simulink library "libturbines"  (Simulink 7.9)
settings: Solver=ode45  StartTime=0.0  StopTime=10.0  RelTol=1e-3
undefined symbols (not defined in the file): DiscIntNeverNeededParam
libraries: simulink x2
settings Model: Creator=grunnet  LastModifiedBy=mikael

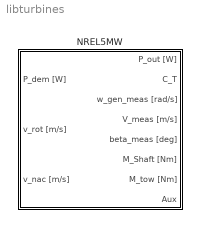
== system libturbines ==
  NREL5MW : Subsystem  mask(Wind Turbine){w_gen_ini=50, beta_ini=0, auto=off, torq_ini=0}
      mask prompts: w_gen_ini "Initial generator velocity  [rad/s]"; beta_ini "Initial blade pitch [degrees]"; auto "Auto initial torque"; torq_ini "Initial generator torque"
      mask help: NREL 5MW Virtual Turbine
      mask init:
      | %l=load(file);
      | l=get_param(gcb,'UserData');
      | env=l.env;
      | wt=l.wt;
      | wt.ctrl.gen.ini=w_gen_ini;
      | 
      | 
      | if(auto)
      |     wt.ctrl.torq.ini=min(interp1(wt.ctrl.torq.wg,wt.ctrl.torq.M,w_gen_ini,'spline'),wt.ctrl.torq.lim);
      | else
      |     wt.ctrl.torq.ini=torq_ini;
      | end
      | 
      | wt.pitch.ini=beta_ini;
      | wt.ctrl.pitch.ini=beta_ini;
      | wt.gen.torq.ini=wt.ctrl.torq.ini;
      | wt.gen.ini=w_gen_ini;
      | wt.rotor.ini=w_gen_ini/wt.gen.N;
      mask Display:
      | image(imread('NREL.png'))
      | 
      | port_label('output',1,'P [W]')
      | port_label('output',2,'CT')
      | port_label('output',3,'w_gen [rad/s]')
      | port_label('output',4,'v_nac [m/s]')
      | port_label('output',5,'pitch [deg]')
      | port_label('output',6,'M_shaft [Nm]')
      | port_label('output',7,'M_tow [Nm]')
      | port_label('output',8,'Aux')
      | 
      | port_label('input',1,'P_max [W]')
      | port_label('input',2,'v_rot [m/s]')
      | port_label('input',3,'v_nac [m/s]')

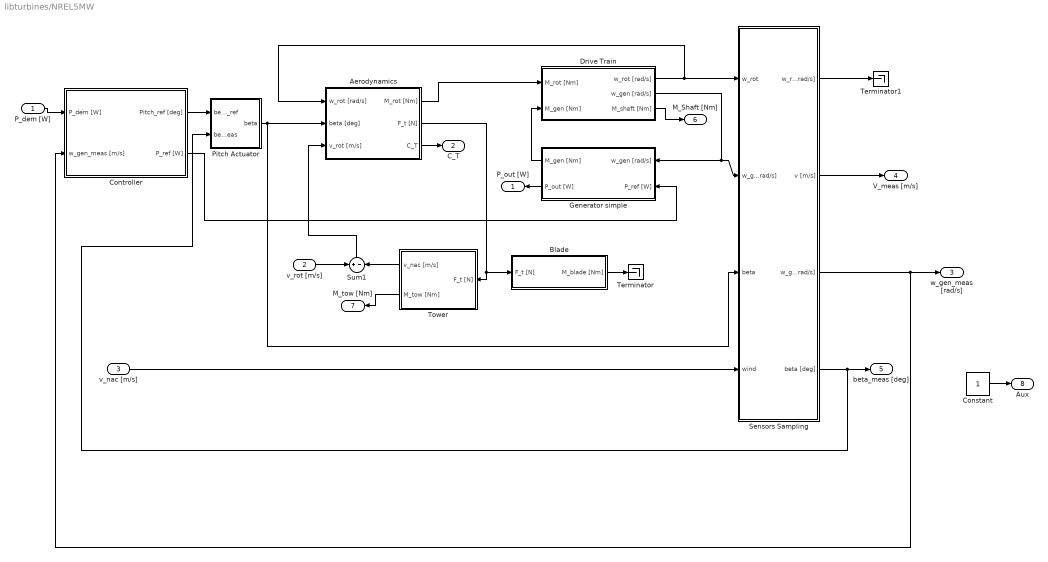
== system libturbines/NREL5MW ==
  P_dem [W] : Inport
  v_rot [m/s] : Inport  Port=2
  v_nac [m/s] : Inport  Port=3
  Aerodynamics : Subsystem
  Blade : Subsystem
  Constant : Constant
  Controller : Subsystem
  Drive Train : Subsystem
  Generator simple : Subsystem
  Pitch Actuator : Subsystem
  Sensors Sampling : Subsystem
  Sum1 : Sum  Inputs=+|-  SaturateOnIntegerOverflow=on  InputSameDT=on  OutDataTypeStr=Inherit: Same as first input
  Terminator : Terminator
  Terminator1 : Terminator
  "Tower " : Subsystem
  P_out [W] : Outport
  C_T : Outport  Port=2
  w_gen_meas [rad/s] : Outport  Port=3
  V_meas [m/s] : Outport  Port=4
  beta_meas [deg] : Outport  Port=5
  M_Shaft [Nm] : Outport  Port=6
  M_tow [Nm] : Outport  Port=7
  Aux : Outport  Port=8
  wires:
  Aerodynamics/3(C_T) -> C_T/1
  Aerodynamics/1(M_rot [Nm]) -> Drive Train/1(M_rot [Nm])
  Drive Train/1(w_rot [rad/s]) -> Sensors Sampling/1("w_rot "), Aerodynamics/1(w_rot [rad/s])
  Generator simple/1(M_gen [Nm]) -> Drive Train/2(M_gen [Nm])
  Drive Train/2(w_gen [rad/s]) -> Generator simple/1(w_gen [rad/s]), Sensors Sampling/2(w_gen [rad/s])
  Sum1/1 -> Aerodynamics/3(v_rot [m/s])
  Sensors Sampling/4(beta [deg]) -> beta_meas [deg]/1, Pitch Actuator/2(beta_meas)
  Sensors Sampling/2(v [m/s]) -> V_meas [m/s]/1
  Controller/2(P_ref [W]) -> Generator simple/2(P_ref [W])
  Sensors Sampling/3(w_gen_meas [rad/s]) -> Controller/2(w_gen_meas [m/s]), w_gen_meas [rad/s]/1
  P_dem [W]/1 -> Controller/1(P_dem [W])
  Controller/1(Pitch_ref [deg]) -> Pitch Actuator/1(beta_ref)
  Pitch Actuator/1(beta) -> Aerodynamics/2(beta [deg]), Sensors Sampling/3(beta)
  "Tower "/1(v_nac [m/s]) -> Sum1/2
  Aerodynamics/2(F_t [N]) -> Blade/1(F_t [N]), "Tower "/1(F_t [N])
  "Tower "/2(M_tow [Nm]) -> M_tow [Nm]/1
  v_rot [m/s]/1 -> Sum1/1
  v_nac [m/s]/1 -> Sensors Sampling/4(wind)
  Generator simple/2(P_out [W]) -> P_out [W]/1
  Drive Train/3(M_shaft [Nm]) -> M_Shaft [Nm]/1
  Blade/1(M_blade [Nm]) -> Terminator/1
  Sensors Sampling/1(w_rot [rad/s]) -> Terminator1/1
  Constant/1 -> Aux/1

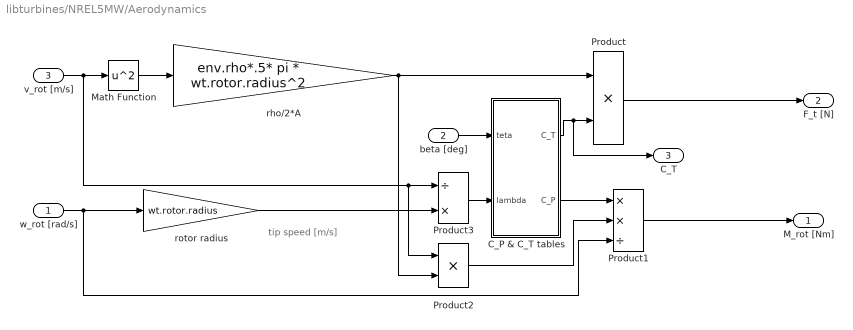
== system libturbines/NREL5MW/Aerodynamics ==
  note: tip speed
      | [m/s]
  w_rot [rad/s] : Inport
  beta [deg] : Inport  Port=2
  v_rot [m/s] : Inport  Port=3
  C_P & C_T tables : Subsystem
  Math Function : Math  Operator=square  SaturateOnIntegerOverflow=on
  Product : Product  SaturateOnIntegerOverflow=on  InputSameDT=on  OutDataTypeStr=Inherit: Same as first input
  Product1 : Product  Inputs=**/  SaturateOnIntegerOverflow=on  InputSameDT=on  OutDataTypeStr=Inherit: Same as first input
  Product2 : Product  SaturateOnIntegerOverflow=on  InputSameDT=on  OutDataTypeStr=Inherit: Same as first input
  Product3 : Product  Inputs=/*  SaturateOnIntegerOverflow=on  InputSameDT=on  OutDataTypeStr=Inherit: Same as first input
  rho/2*A : Gain  Gain=env.rho*.5* pi * wt.rotor.radius^2  SaturateOnIntegerOverflow=on  OutDataTypeStr=Inherit: Same as input  ParamDataTypeStr=Inherit: Same as input
  rotor radius : Gain  Gain=wt.rotor.radius  SaturateOnIntegerOverflow=on  OutDataTypeStr=Inherit: Same as input  ParamDataTypeStr=Inherit: Same as input
  M_rot [Nm] : Outport
  F_t [N] : Outport  Port=2
  C_T : Outport  Port=3
  wires:
  rho/2*A/1 -> Product2/2, Product/1
  w_rot [rad/s]/1 -> rotor radius/1, Product1/3
  Product/1 -> F_t [N]/1
  rotor radius/1 -> Product3/2
  v_rot [m/s]/1 -> Math Function/1, Product3/1, Product2/1
  Math Function/1 -> rho/2*A/1
  beta [deg]/1 -> C_P & C_T tables/1(teta)
  C_P & C_T tables/1(C_T) -> Product/2, C_T/1
  C_P & C_T tables/2(C_P) -> Product1/1
  Product2/1 -> Product1/2
  Product3/1 -> C_P & C_T tables/2(lambda)
  Product1/1 -> M_rot [Nm]/1

== system libturbines/NREL5MW/Blade ==
  F_t [N] : Inport
  1/3*Fb*2*r : Gain  Gain=1/3*wt.rotor.radius*2  SaturateOnIntegerOverflow=on  OutDataTypeStr=Inherit: Same as input  ParamDataTypeStr=Inherit: Same as input
  M_blade [Nm] : Outport
  wires:
  1/3*Fb*2*r/1 -> M_blade [Nm]/1
  F_t [N]/1 -> 1/3*Fb*2*r/1

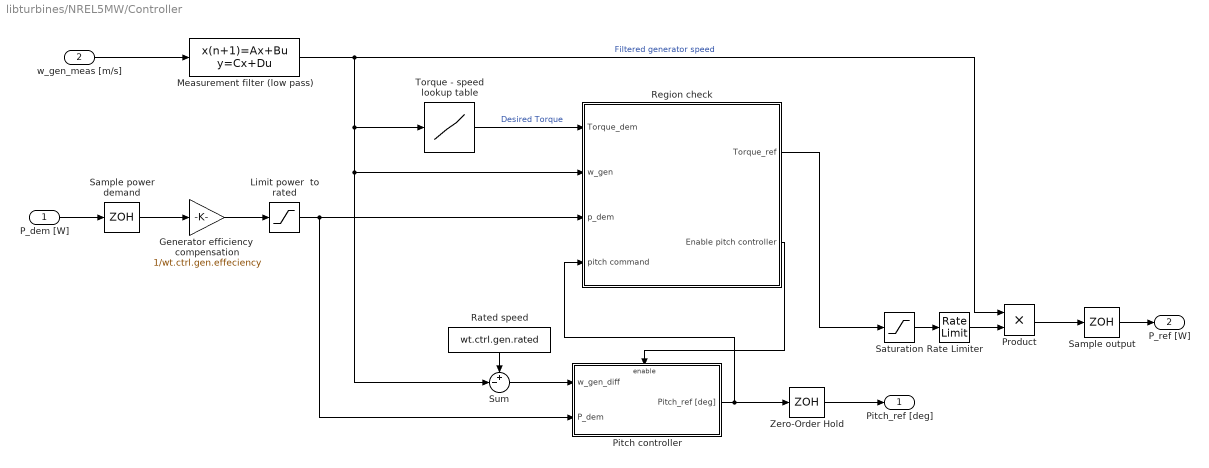
== system libturbines/NREL5MW/Controller ==
  P_dem [W] : Inport
  w_gen_meas [m/s] : Inport  Port=2
  Generator efficiency  compensation : Gain  Gain=1/wt.ctrl.gen.effeciency
  Limit power  to rated : Saturate  UpperLimit=wt.ctrl.p_rated  LowerLimit=0
  Measurement filter (low pass) : DiscreteStateSpace  A=wt.ctrl.alpha  B=1-wt.ctrl.alpha  C=wt.ctrl.alpha  D=1-wt.ctrl.alpha  X0=wt.ctrl.gen.ini  SampleTime=wt.ctrl.Ts
  Pitch controller : Subsystem  TreatAsAtomicUnit=on
  Product : Product  RndMeth=Zero
  Rate Limiter : RateLimiter  RisingSlewLimit=wt.ctrl.torq.ratelim  FallingSlewLimit=-wt.ctrl.torq.ratelim  SampleTimeMode=inherited  InitialCondition=wt.ctrl.torq.ini
  Rated speed : Constant  Value=wt.ctrl.gen.rated
  Region check : Subsystem
  Sample output : ZeroOrderHold  SampleTime=wt.ctrl.Ts
  Sample power demand : ZeroOrderHold  SampleTime=wt.ctrl.Ts
  Saturation : Saturate  UpperLimit=wt.ctrl.torq.lim  LowerLimit=0
  Sum : Sum  Inputs=+-|
  Torque - speed lookup table : Lookup  InputValues=wt.ctrl.torq.wg  Table=wt.ctrl.torq.M  LookUpMeth=Interpolation-Use End Values
  Zero-Order Hold : ZeroOrderHold  SampleTime=wt.ctrl.Ts
  Pitch_ref [deg] : Outport
  P_ref [W] : Outport  Port=2
  wires:
  w_gen_meas [m/s]/1 -> Measurement filter (low pass)/1
  Measurement filter (low pass)/1 -> Product/1, Torque - speed lookup table/1, Region check/2(w_gen), Sum/2  "Filtered generator speed"
  Saturation/1 -> Rate Limiter/1
  Rate Limiter/1 -> Product/2
  Pitch controller/1(Pitch_ref [deg]) -> Zero-Order Hold/1, Region check/4(pitch command)
  Torque - speed lookup table/1 -> Region check/1(Torque_dem)  "Desired Torque"
  P_dem [W]/1 -> Sample power demand/1
  Region check/1(Torque_ref) -> Saturation/1
  Limit power  to rated/1 -> Pitch controller/2(P_dem), Region check/3(p_dem)
  Zero-Order Hold/1 -> Pitch_ref [deg]/1
  Sample output/1 -> P_ref [W]/1
  Generator efficiency  compensation/1 -> Limit power  to rated/1
  Product/1 -> Sample output/1
  Sample power demand/1 -> Generator efficiency  compensation/1
  Rated speed/1 -> Sum/1
  Sum/1 -> Pitch controller/1(w_gen_diff)
  Region check/2(Enable pitch controller) -> Pitch controller/Enable

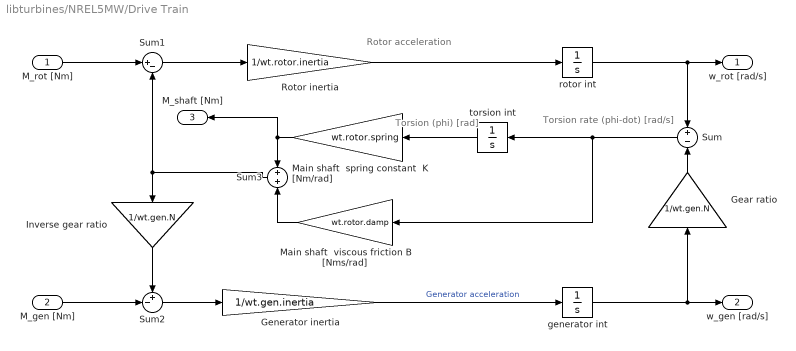
== system libturbines/NREL5MW/Drive Train ==
  note: Torsion rate (phi-dot) [rad/s]
  note: Torsion (phi)
      | [rad]
  note: Rotor acceleration
  M_rot [Nm] : Inport
  M_gen [Nm] : Inport  Port=2
  Gear ratio : Gain  Gain=1/wt.gen.N
  Generator inertia : Gain  Gain=1/wt.gen.inertia
  Inverse gear ratio : Gain  Gain=1/wt.gen.N
  Main shaft  spring constant  K [Nm/rad] : Gain  Gain=wt.rotor.spring
  Main shaft  viscous friction B [Nms/rad] : Gain  Gain=wt.rotor.damp
  Rotor inertia : Gain  Gain=1/wt.rotor.inertia
  Sum : Sum  Inputs=+|-
  Sum1 : Sum  Inputs=|+-
  Sum2 : Sum  Inputs=+-|
  Sum3 : Sum  Inputs=+|+
  generator int : Integrator  InitialCondition=wt.gen.ini
  rotor int : Integrator  InitialCondition=wt.rotor.ini
  torsion int : Integrator
  w_rot [rad/s] : Outport
  w_gen [rad/s] : Outport  Port=2
  M_shaft [Nm] : Outport  Port=3
  wires:
  M_rot [Nm]/1 -> Sum1/1
  rotor int/1 -> w_rot [rad/s]/1, Sum/1
  generator int/1 -> w_gen [rad/s]/1, Gear ratio/1
  Gear ratio/1 -> Sum/2
  Sum/1 -> torsion int/1, Main shaft  viscous friction B [Nms/rad]/1
  torsion int/1 -> Main shaft  spring constant  K [Nm/rad]/1
  Main shaft  spring constant  K [Nm/rad]/1 -> Sum3/1, M_shaft [Nm]/1
  Main shaft  viscous friction B [Nms/rad]/1 -> Sum3/2
  M_gen [Nm]/1 -> Sum2/2
  Sum3/1 -> Inverse gear ratio/1, Sum1/2
  Inverse gear ratio/1 -> Sum2/1
  Sum2/1 -> Generator inertia/1
  Sum1/1 -> Rotor inertia/1
  Rotor inertia/1 -> rotor int/1
  Generator inertia/1 -> generator int/1  "Generator acceleration"

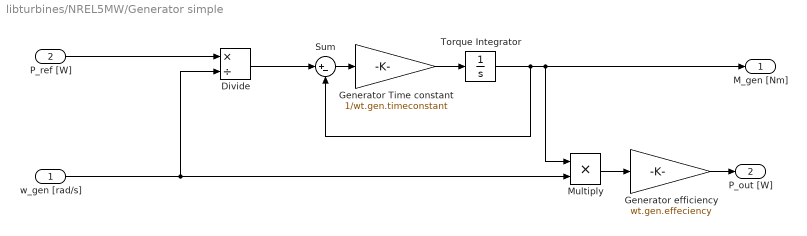
== system libturbines/NREL5MW/Generator simple ==
  w_gen [rad/s] : Inport
  P_ref [W] : Inport  Port=2
  Divide : Product  Inputs=*/
  Generator Time constant : Gain  Gain=1/wt.gen.timeconstant
  Generator efficiency : Gain  Gain=wt.gen.effeciency
  Multiply : Product  Inputs=**
  Sum : Sum  Inputs=|+-
  Torque Integrator : Integrator  InitialCondition=wt.gen.torq.ini
  M_gen [Nm] : Outport
  P_out [W] : Outport  Port=2
  wires:
  P_ref [W]/1 -> Divide/1
  w_gen [rad/s]/1 -> Divide/2, Multiply/2
  Torque Integrator/1 -> Sum/2, Multiply/1, M_gen [Nm]/1
  Divide/1 -> Sum/1
  Multiply/1 -> Generator efficiency/1
  Generator efficiency/1 -> P_out [W]/1
  Generator Time constant/1 -> Torque Integrator/1
  Sum/1 -> Generator Time constant/1

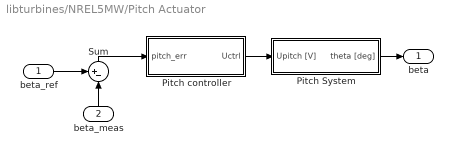
== system libturbines/NREL5MW/Pitch Actuator ==
  beta_ref : Inport
  beta_meas : Inport  Port=2
  Pitch System : Subsystem
  Pitch controller : Subsystem
  Sum : Sum  Inputs=+-|  SaturateOnIntegerOverflow=on  InputSameDT=on  OutDataTypeStr=Inherit: Same as first input
  beta : Outport
  wires:
  Pitch controller/1(Uctrl) -> Pitch System/1(Upitch [V])
  Sum/1 -> Pitch controller/1(pitch_err)
  beta_ref/1 -> Sum/1
  Pitch System/1(theta [deg]) -> beta/1
  beta_meas/1 -> Sum/2

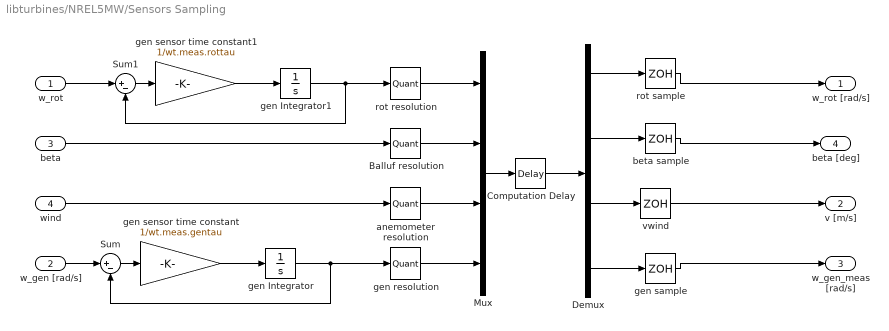
== system libturbines/NREL5MW/Sensors Sampling ==
  "w_rot " : Inport
  w_gen [rad/s] : Inport  Port=2
  beta : Inport  Port=3
  wind : Inport  Port=4
  Balluf resolution : Quantizer  QuantizationInterval=wt.meas.ballufres
  Computation Delay : TransportDelay  DelayTime=wt.meas.delay  InitialOutput=[wt.rotor.ini wt.pitch.ini 0 wt.gen.ini]
  Demux : Demux
  Mux : Mux
  Sum : Sum  Inputs=|+-
  Sum1 : Sum  Inputs=|+-
  anemometer resolution : Quantizer  QuantizationInterval=wt.meas.aneres
  beta sample : ZeroOrderHold  SampleTime=wt.meas.Ts
  gen Integrator : Integrator  InitialCondition=wt.gen.ini
  gen Integrator1 : Integrator  InitialCondition=wt.rotor.ini
  gen resolution : Quantizer  QuantizationInterval=wt.meas.genres
  gen sample : ZeroOrderHold  SampleTime=wt.meas.Ts
  gen sensor time constant : Gain  Gain=1/wt.meas.gentau
  gen sensor time constant1 : Gain  Gain=1/wt.meas.rottau
  rot resolution : Quantizer  QuantizationInterval=wt.meas.rotres
  rot sample : ZeroOrderHold  SampleTime=wt.meas.Ts
  vwind : ZeroOrderHold  SampleTime=wt.meas.Ts
  w_rot [rad/s] : Outport  InitialOutput=0
  v [m/s] : Outport  Port=2  InitialOutput=0
  w_gen_meas [rad/s] : Outport  Port=3  InitialOutput=0
  beta [deg] : Outport  Port=4  InitialOutput=0
  wires:
  "w_rot "/1 -> Sum1/1
  gen Integrator1/1 -> rot resolution/1, Sum1/2
  gen sensor time constant1/1 -> gen Integrator1/1
  Sum1/1 -> gen sensor time constant1/1
  gen Integrator/1 -> gen resolution/1, Sum/2
  gen sensor time constant/1 -> gen Integrator/1
  Sum/1 -> gen sensor time constant/1
  vwind/1 -> v [m/s]/1
  Demux/3 -> vwind/1
  Demux/2 -> beta sample/1
  Computation Delay/1 -> Demux/1
  beta sample/1 -> beta [deg]/1
  rot sample/1 -> w_rot [rad/s]/1
  Demux/1 -> rot sample/1
  beta/1 -> Balluf resolution/1
  Mux/1 -> Computation Delay/1
  wind/1 -> anemometer resolution/1
  rot resolution/1 -> Mux/1
  Balluf resolution/1 -> Mux/2
  anemometer resolution/1 -> Mux/3
  gen sample/1 -> w_gen_meas [rad/s]/1
  Demux/4 -> gen sample/1
  w_gen [rad/s]/1 -> Sum/1
  gen resolution/1 -> Mux/4

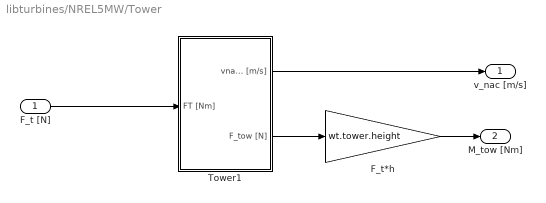
== system libturbines/NREL5MW/Tower  ==
  F_t [N] : Inport
  F_t*h : Gain  Gain=wt.tower.height  SaturateOnIntegerOverflow=on  OutDataTypeStr=Inherit: Same as input  ParamDataTypeStr=Inherit: Same as input
  Tower1 : Subsystem  mask(Tower (thrustwise)){mtop=wt.top.mass, mtow=wt.tower.mass, ftowY=wt.tower.eigfreq, dampY=wt.tower.damp}
      mask prompts: mtop "Mass of towertop [kg]"; mtow "Aequivalent tower mass [kg]"; ftowY "Tower eigenfrequency [Hz]"; dampY "Damping coefficient"
      mask help: Thrustwise dynamics of the tower
      mask init:
      | A = [-4*pi*dampY*ftowY,  -4*pi^2*ftowY^2  ; ...
      |                     1                               0       ];
      | B = [1/(mtop+mtow) ; ...
      |           0];
      | C = [1 0 ; ...
      |     0 -4*pi^2*ftowY^2*(mtop+mtow)];
      | D = zeros(2,1);
      mask Help: The thrustwise tower dynamics are modelled as a linear oscillator
  v_nac [m/s] : Outport
  M_tow [Nm] : Outport  Port=2
  wires:
  Tower1/1(vnac [m/s]) -> v_nac [m/s]/1
  F_t [N]/1 -> Tower1/1(FT [Nm])
  F_t*h/1 -> M_tow [Nm]/1
  Tower1/2(F_tow [N]) -> F_t*h/1

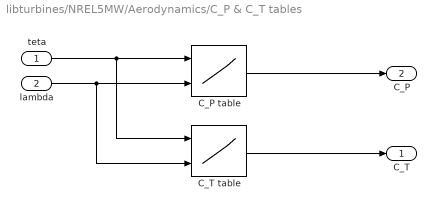
== system libturbines/NREL5MW/Aerodynamics/C_P & C_T tables ==
  teta : Inport
  lambda : Inport  Port=2
  "C_P table " : Lookup2D  RowIndex=wt.cp.beta  ColumnIndex=wt.cp.tsr  Table=wt.cp.table  LookUpMeth=Interpolation-Use End Values  SaturateOnIntegerOverflow=on  InputSameDT=on
  C_T table : Lookup2D  RowIndex=wt.ct.beta  ColumnIndex=wt.ct.tsr  Table=wt.ct.table  LookUpMeth=Interpolation-Use End Values  SaturateOnIntegerOverflow=on  InputSameDT=on
  C_T : Outport
  C_P : Outport  Port=2
  wires:
  lambda/1 -> "C_P table "/2, C_T table/2
  teta/1 -> "C_P table "/1, C_T table/1
  "C_P table "/1 -> C_P/1
  C_T table/1 -> C_T/1

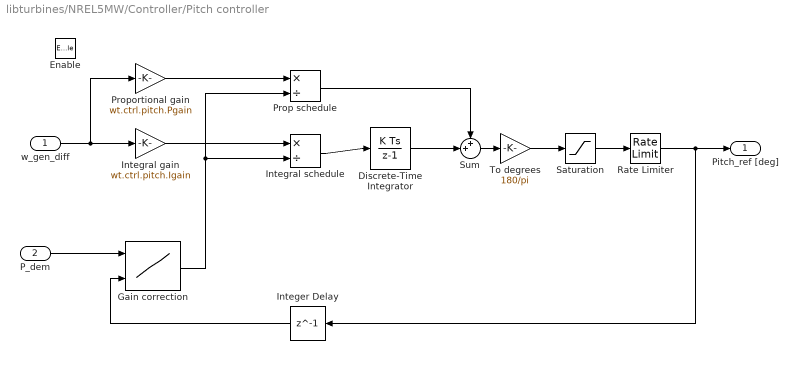
== system libturbines/NREL5MW/Controller/Pitch controller ==
  w_gen_diff : Inport
  P_dem : Inport  Port=2
  Enable : EnablePort  StatesWhenEnabling=reset  PropagateVarSize=During execution
  Discrete-Time Integrator : DiscreteIntegrator  SampleTime=wt.ctrl.Ts  LimitOutput=on  UpperSaturationLimit=wt.ctrl.pitch.ulim*pi/180  LowerSaturationLimit=wt.ctrl.pitch.llim  ICPrevOutput=DiscIntNeverNeededParam  ICPrevScaledInput=DiscIntNeverNeededParam
  Gain correction : Lookup2D  RowIndex=wt.ctrl.pitch.pwr  ColumnIndex=wt.ctrl.pitch.beta  Table=wt.ctrl.pitch.gs  LookUpMeth=Interpolation-Use End Values
  Integer Delay : Delay  DelayLength=1  InputProcessing=Inherited
  Integral gain : Gain  Gain=wt.ctrl.pitch.Igain
  Integral schedule : Product  Inputs=*/  RndMeth=Zero
  Prop schedule : Product  Inputs=*/  RndMeth=Zero
  Proportional gain : Gain  Gain=wt.ctrl.pitch.Pgain
  Rate Limiter : RateLimiter  RisingSlewLimit=wt.ctrl.pitch.ratelim  FallingSlewLimit=-wt.ctrl.pitch.ratelim  SampleTimeMode=inherited  InitialCondition=wt.ctrl.pitch.ini
  Saturation : Saturate  UpperLimit=wt.ctrl.pitch.ulim  LowerLimit=0
  Sum : Sum  Inputs=++|
  To degrees : Gain  Gain=180/pi
  Pitch_ref [deg] : Outport  OutputWhenDisabled=reset  InitialOutput=wt.ctrl.torq.beta
  wires:
  Saturation/1 -> Rate Limiter/1
  Rate Limiter/1 -> Pitch_ref [deg]/1, Integer Delay/1
  Integral schedule/1 -> Discrete-Time Integrator/1
  Gain correction/1 -> Prop schedule/2, Integral schedule/2
  Sum/1 -> To degrees/1
  Discrete-Time Integrator/1 -> Sum/2
  Proportional gain/1 -> Prop schedule/1
  Prop schedule/1 -> Sum/1
  Integral gain/1 -> Integral schedule/1
  w_gen_diff/1 -> Proportional gain/1, Integral gain/1
  To degrees/1 -> Saturation/1
  Integer Delay/1 -> Gain correction/2
  P_dem/1 -> Gain correction/1

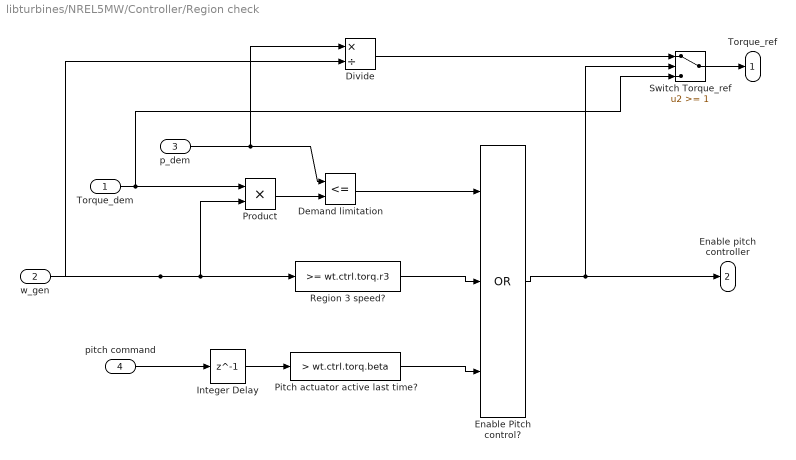
== system libturbines/NREL5MW/Controller/Region check ==
  Torque_dem : Inport
  w_gen : Inport  Port=2
  p_dem : Inport  Port=3
  pitch command : Inport  Port=4
  Demand limitation : RelationalOperator  Operator=<=  OutDataTypeStr=boolean
  Divide : Product  Inputs=*/
  Enable Pitch control? : Logic  Operator=OR  Inputs=3  AllPortsSameDT=off  OutDataTypeStr=boolean
  Integer Delay : Delay  DelayLength=1  InputProcessing=Inherited
  Pitch actuator active last time? : simulink/Logic and Bit Operations/Compare To Constant  relop=>  const=wt.ctrl.torq.beta  OutDataTypeStr=uint8  ZeroCross=off
  Product : Product  RndMeth=Zero
  Region 3 speed? : simulink/Logic and Bit Operations/Compare To Constant  relop=>=  const=wt.ctrl.torq.r3  OutDataTypeStr=uint8  ZeroCross=off
  Switch Torque_ref : Switch  Threshold=1
  Torque_ref : Outport
  Enable pitch controller : Outport  Port=2
  wires:
  pitch command/1 -> Integer Delay/1
  w_gen/1 -> Product/2, Region 3 speed?/1, Divide/2
  Pitch actuator active last time?/1 -> Enable Pitch control?/3
  Region 3 speed?/1 -> Enable Pitch control?/2
  Integer Delay/1 -> Pitch actuator active last time?/1
  Enable Pitch control?/1 -> Enable pitch controller/1, Switch Torque_ref/2
  Product/1 -> Demand limitation/2
  Torque_dem/1 -> Product/1, Switch Torque_ref/3
  p_dem/1 -> Divide/1, Demand limitation/1
  Demand limitation/1 -> Enable Pitch control?/1
  Switch Torque_ref/1 -> Torque_ref/1
  Divide/1 -> Switch Torque_ref/1

== system libturbines/NREL5MW/Pitch Actuator/Pitch System ==
  Upitch [V] : Inport
  Hydraulic delay time : TransportDelay  DelayTime=wt.pitch.delay
  Hydraulic  time constant : TransferFcn  Denominator=[wt.pitch.tau 1]
  Integrator : Integrator  InitialCondition=wt.pitch.ini
  theta [deg] : Outport
  wires:
  Upitch [V]/1 -> Hydraulic delay time/1
  Integrator/1 -> theta [deg]/1
  Hydraulic delay time/1 -> Hydraulic  time constant/1
  Hydraulic  time constant/1 -> Integrator/1

== system libturbines/NREL5MW/Pitch Actuator/Pitch controller ==
  pitch_err : Inport
  e.k : Gain  Gain=wt.pitch.K  SaturateOnIntegerOverflow=on  OutDataTypeStr=Inherit: Same as input  ParamDataTypeStr=Inherit: Same as input
  Uctrl : Outport
  wires:
  e.k/1 -> Uctrl/1
  pitch_err/1 -> e.k/1

== system libturbines/NREL5MW/Tower /Tower1 ==
  FT [Nm] : Inport
  Demux : Demux  Outputs=2
  Tower : StateSpace  A=A  B=B  C=C  D=D  X0=zeros(2,1)
  vnac [m/s] : Outport  InitialOutput=0
  F_tow [N] : Outport  Port=2  InitialOutput=0
  wires:
  Tower/1 -> Demux/1
  Demux/1 -> vnac [m/s]/1
  FT [Nm]/1 -> Tower/1
  Demux/2 -> F_tow [N]/1
